simulink model "Equaliser 1"  (R2024b)
settings: Solver=VariableStepAuto  StartTime=0.0  StopTime=10.0  RelTol=1e-3
undefined symbols (not defined in the file): doppler, pskmod
libraries: commchan3 x4, commdigbbndpm3 x4, commsink2 x2, dspxfrm3 x2, simulink x1, commeq3 x1, commrandsrc3 x1
settings Model: Creator=anaht  LastModifiedBy=anaht

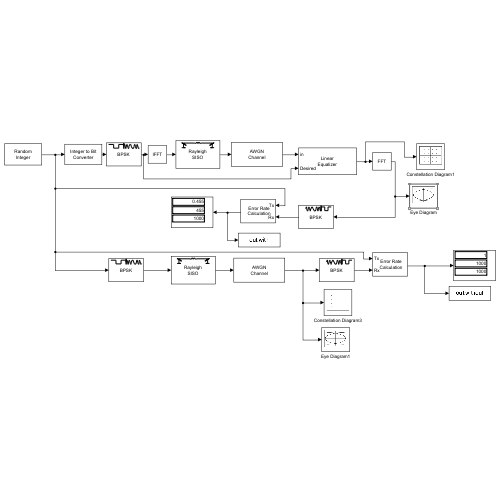
[thumbnail: Simulink's stored preview of the top-level diagram]
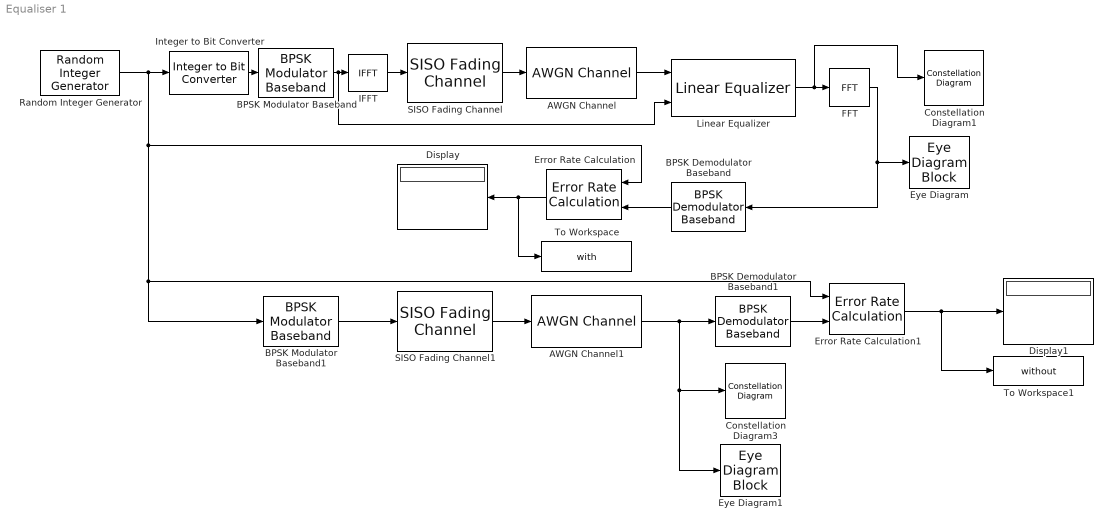
== system Equaliser 1 ==
  AWGN Channel : commchan3/AWGN Channel  LegacyMode=off  NoiseMethod="Signal to noise ratio  (Eb/No)"  noiseMode="Signal to noise ratio  (SNR)"  EbNo=20  EsNo=10  SNR=10  BitsPerSymbol=1  SignalPower=1  SamplesPerSymbol=1  SymbolPeriod=1  VarianceSource=Parameter  Variance=1  RandomStream=Global stream  Seed=67  SimulateUsing=Code generation
  AWGN Channel1 : commchan3/AWGN Channel  LegacyMode=off  NoiseMethod="Signal to noise ratio  (Eb/No)"  noiseMode="Signal to noise ratio  (SNR)"  EbNo=20  EsNo=10  SNR=10  BitsPerSymbol=1  SignalPower=1  SamplesPerSymbol=1  SymbolPeriod=1  VarianceSource=Parameter  Variance=1  RandomStream=Global stream  Seed=67  SimulateUsing=Code generation
  BPSK Demodulator Baseband : commdigbbndpm3/BPSK Demodulator Baseband  DecType=Hard decision  VarSource=Dialog  Variance=1  Ph=0  outDtype=Inherit via internal rule  derotateFactorWordLen=16  derotateFactorDataTypeStr=Inherit: Same word length as input  derotateFactorLastDataTypeStr=Inherit: Same word length as input
      settings: LibrarySourceBlock=|
      | commhdldigbbndpm/BPSK
      | Demodulator
      | Baseband
  BPSK Demodulator Baseband1 : commdigbbndpm3/BPSK Demodulator Baseband  DecType=Hard decision  VarSource=Dialog  Variance=1  Ph=0  outDtype=Inherit via internal rule  derotateFactorWordLen=16  derotateFactorDataTypeStr=Inherit: Same word length as input  derotateFactorLastDataTypeStr=Inherit: Same word length as input
      settings: LibrarySourceBlock=|
      | commhdldigbbndpm/BPSK
      | Demodulator
      | Baseband
  BPSK Modulator Baseband : commdigbbndpm3/BPSK Modulator Baseband  Ph=0  outDtype=double  outWordLen=16  outUDDataType=sfix(16)  outFracLenMode=Best precision  outFracLen=15  outDataTypeStr=double  outLastDataTypeStr=double
  BPSK Modulator Baseband1 : commdigbbndpm3/BPSK Modulator Baseband  Ph=0  outDtype=double  outWordLen=16  outUDDataType=sfix(16)  outFracLenMode=Best precision  outFracLen=15  outDataTypeStr=double  outLastDataTypeStr=double
  Constellation Diagram1 : ConstellationDiagram  WindowPosition=[340.000000,60.000000,600.000000,600.000000,]  ScopeFrameLocation=window  ReferenceConstellation=BPSK  XLimits=[-0.3647637597163798,0.4937300882632287]  YLimits=[-0.3647637597163798,0.4937300882632287]
  Constellation Diagram3 : ConstellationDiagram  WindowPosition=[340.000000,60.000000,600.000000,600.000000,]  ScopeFrameLocation=window  ReferenceConstellation=BPSK  XLimits=[-17.256527572771475,14.306800618258467]  YLimits=[-17.256527572771475,14.306800618258467]
  Display : Display
  Display1 : Display
  Error Rate Calculation : commsink2/Error Rate Calculation  N=0  st_delay=0  cp_mode=Entire frame  subframe=[]  PMode=Port  WsName=ErrorVec  RsMode2=off  stop=off  numErr=100  maxBits=1e6
  Error Rate Calculation1 : commsink2/Error Rate Calculation  N=0  st_delay=0  cp_mode=Entire frame  subframe=[]  PMode=Port  WsName=ErrorVec  RsMode2=off  stop=off  numErr=100  maxBits=1e6
  Eye Diagram : EyeDiagramBlock  WindowPosition=[240.000000,110.000000,800.000000,500.000000,]  ScopeFrameLocation=window  SamplesPerSymbol=1
  Eye Diagram1 : EyeDiagramBlock  WindowPosition=[240.000000,110.000000,800.000000,500.000000,]  ScopeFrameLocation=window  SamplesPerSymbol=1  YLimits=[-1.7947969217938031,1.7968264894383947]
  FFT : dspxfrm3/FFT  FFTImplementation=Auto  CompMethod=Table lookup  TableOpt=NEW  TableOptActive=Speed  BitRevOrder=off  Normalize=off  InheritFFTLength=on  FFTLength=64  WrapInput=on  roundingMode=Ceiling  overflowMode=off  firstCoeffDataTypeStr=Inherit: Same word length as input  firstCoeffLastDataTypeStr=Inherit: Same word length as input  outputMin=[]  outputMax=[]
  IFFT : dspxfrm3/IFFT  FFTImplementation=Auto  CompMethod=Table lookup  TableOpt=NEW  TableOptActive=Speed  BitRevOrder=off  cs_in=off  Normalize=on  InheritFFTLength=on  FFTLength=64  WrapInput=on  mode=Real  outSamplingMode=Sample based  roundingMode=Ceiling  overflowMode=off  firstCoeffDataTypeStr=Inherit: Same word length as input  firstCoeffLastDataTypeStr=Inherit: Same word length as input  outputMin=[]  outputMax=[]
  Integer to Bit Converter : simulink/Logic and Bit Operations/Integer to Bit Converter  nbits=1  signedInputValues=Unsigned  bitOrder=MSB first  outDtype=Inherit via internal rule
  Linear Equalizer : commeq3/Linear Equalizer  NumTaps=5  Constellation=pskmod( 0:3, 4, pi/4, 'bin' )  InputSamplesPerSymbol=1  Algorithm=LMS  StepSize=0.01  ForgettingFactor=0.99  InitialInverseCorrelationMatrix=0.1  ReferenceTap=3  InputDelay=0  AdaptWeightsSource=Property  AdaptWeights=on  InitialWeightsSource=Auto  InitialWeights=0  TrainingInitialWeights=0  BlindInitialWeights=[ 0; 0; 1; 0; 0 ]  WeightUpdatePeriod=1  TrainingFlagInputPort=off  AdaptAfterTraining=on  ResetInputPort=off  ErrorOutputPort=off  TapWeightsOutputPort=off  SimulateUsing=Code generation
  Random Integer Generator : commrandsrc3/Random Integer Generator  SetSize=2  SeedSource=Auto  Seed=0  SampleTime=1  SamplesPerFrame=1000  OutputDataType=double  SimulateUsing=Interpreted execution
  SISO Fading Channel : commchan3/SISO Fading Channel  InheritSampleRate=on  SampleRate=1  PathDelays=0  AveragePathGains=0  NormalizePathGains=on  FadingDistribution=Rayleigh  KFactor=25  DirectPathDopplerShift=0  DirectPathInitialPhase=0  MaximumDopplerShift=0.0001  DopplerSpectrum=doppler('Jakes')  RandomStream=mt19937ar with seed  Seed=73  PathGainsOutputPort=off  ChannelFilterDelayOutputPort=off  SimulateUsing=Interpreted execution  Visualization=Off  PathsForDopplerDisplay=1  SamplesToDisplay=25%
  SISO Fading Channel1 : commchan3/SISO Fading Channel  InheritSampleRate=on  SampleRate=1  PathDelays=0  AveragePathGains=0  NormalizePathGains=on  FadingDistribution=Rayleigh  KFactor=25  DirectPathDopplerShift=0  DirectPathInitialPhase=0  MaximumDopplerShift=0.0001  DopplerSpectrum=doppler('Jakes')  RandomStream=mt19937ar with seed  Seed=73  PathGainsOutputPort=off  ChannelFilterDelayOutputPort=off  SimulateUsing=Interpreted execution  Visualization=Off  PathsForDopplerDisplay=1  SamplesToDisplay=25%
  To Workspace : ToWorkspace  VariableName=with  SampleTime=-1
      settings: Save2DSignal=2-D array (concatenate along first dimension)
  To Workspace1 : ToWorkspace  VariableName=without  SampleTime=-1
      settings: Save2DSignal=2-D array (concatenate along first dimension)
  wires:
  AWGN Channel/1 -> Linear Equalizer/1
  BPSK Demodulator Baseband/1 -> Error Rate Calculation/2
  Error Rate Calculation/1 -> To Workspace/1, Display/1
  SISO Fading Channel1/1 -> AWGN Channel1/1
  BPSK Modulator Baseband1/1 -> SISO Fading Channel1/1
  BPSK Demodulator Baseband1/1 -> Error Rate Calculation1/2
  Error Rate Calculation1/1 -> To Workspace1/1, Display1/1
  FFT/1 -> Eye Diagram/1, BPSK Demodulator Baseband/1
  SISO Fading Channel/1 -> AWGN Channel/1
  IFFT/1 -> SISO Fading Channel/1
  Linear Equalizer/1 -> Constellation Diagram1/1, FFT/1
  Random Integer Generator/1 -> Integer to Bit Converter/1, Error Rate Calculation/1, Error Rate Calculation1/1, BPSK Modulator Baseband1/1
  AWGN Channel1/1 -> Eye Diagram1/1, Constellation Diagram3/1, BPSK Demodulator Baseband1/1
  Integer to Bit Converter/1 -> BPSK Modulator Baseband/1
  BPSK Modulator Baseband/1 -> Linear Equalizer/2, IFFT/1
